simulink model "hcci_eng_with_delay"  (R2018a)
settings: Solver=VariableStepAuto  StartTime=0.0  StopTime=t_end  RelTol=1e-3
values from neighbouring files (symbols this model uses):
  A01 = f(90)    [load_param.m]
  A20 = f(70)    [load_param.m]
  A21 = f(50)    [load_param.m]
  AFR_EGO_0 = AFR_s    (= 20)    [load_param.m]
  AFR_s = 20    [load_param.m]
  alpha_1 = 0.752    [load_param.m]
  alpha_2 = -0.180    (= -0.18)    [load_param.m]
  alpha_3 = 0.015    [load_param.m]
  b1_0 = 0    [load_param.m]
  b2_0 = 0    [load_param.m]
  beta_0 = 1.035    [load_param.m]
  beta_1 = 1.1568    [load_param.m]
  dT_er2 = 75    [load_param.m]
  gamma = 1.4    [load_param.m]
  kappa_0 = -2.2107    [load_param.m]
  kappa_1 = 61.5556    [load_param.m]
  kappa_2 = 4.6052    [load_param.m]
  kappa_3 = 0.964    [load_param.m]
  m1_0 = p0*V1/(R*T1)    (= 1.2204509185e-06)    [load_param.m]
  m2_0 = p0*V2/(R*T1)    (= 1.40821259827e-05)    [load_param.m]
  N = 1000    [load_param.m]
  p0 = 101    [load_param.m]
  p2_0 = p0    (= 101)    [load_param.m]
  R = 296.25    [AR_solver_tester.m]    (also in HCCI_Combustion.m; combustion_param.m; load_param.m; testor.m)
  T1 = 90 + 273.15    (= 363.15)    [load_param.m]
  tau = 120 / N    (= 0.12)    [load_param.m]
  tau_EGO = 0.08    [load_param.m]
  u_rbl = 2    [load_param.m]
  V1 = 0.0013    [load_param.m]
  V2 = 0.015    [load_param.m]
  V_ivc = V_d + V_TDC    (= 0.000592307692308)    [AR_solver_tester.m]    (also in HCCI_Combustion.m = double(subs(Vc, theta, theta_ivc)); load_eng.m = double(subs(Vc, theta, theta_ivc)); load_param.m; testor.m = double(subs(Vc, theta, theta_ivc)))
  Wf = 11.9e-3    (= 0.0119)    [load_param.m]
undefined symbols (not defined in the file or in its folder): C_d
settings Model: Creator=Lenovo  LastModifiedBy=Lenovo

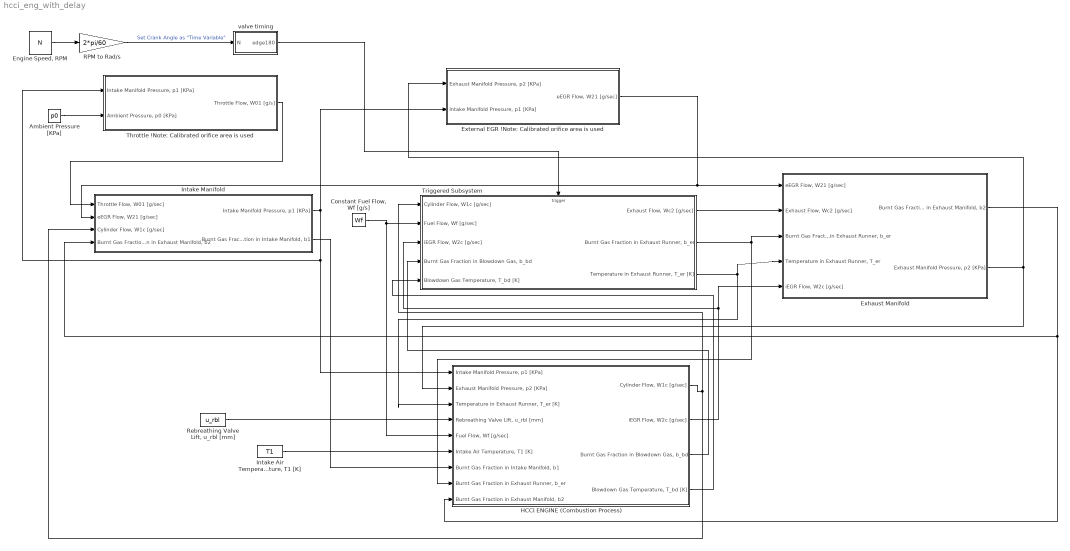
== system hcci_eng_with_delay ==
  Ambient Pressure [KPa] : Constant  Value=p0
  "Constant Fuel Flow, Wf [g/s] " : Constant  Value=Wf
  "Engine Speed, RPM" : Constant  Value=N
  Exhaust Manifold : Subsystem
  "External EGR !Note: Calibrated orifice area is used " : Subsystem
  HCCI ENGINE (Combustion Process) : Subsystem
  "Intake Air Temperature, T1 [K]" : Constant  Value=T1
  Intake Manifold : Subsystem
  RPM to Rad/s : Gain  Gain=2*pi/60
  "Rebreathing Valve Lift, u_rbl [mm]" : Constant  Value=u_rbl
  Throttle !Note: Calibrated orifice area is used : Subsystem
  Triggered Subsystem : Subsystem  TreatAsAtomicUnit=on
  valve timing : Subsystem
  wires:
  "Engine Speed, RPM"/1 -> RPM to Rad/s/1
  Ambient Pressure [KPa]/1 -> Throttle !Note: Calibrated orifice area is used/2("Ambient Pressure, p0 [KPa]")
  Throttle !Note: Calibrated orifice area is used/1("Throttle Flow, W01 [g/s]") -> Intake Manifold/1("Throttle Flow, W01 [g/sec]")
  Intake Manifold/1("Intake Manifold Pressure, p1 [KPa]") -> "External EGR !Note: Calibrated orifice area is used "/2("Intake Manifold Pressure, p1 [KPa]"), HCCI ENGINE (Combustion Process)/1("Intake Manifold Pressure, p1 [KPa]"), Throttle !Note: Calibrated orifice area is used/1("Intake Manifold Pressure, p1 [KPa]")
  "External EGR !Note: Calibrated orifice area is used "/1("eEGR Flow, W21 [g/sec]") -> Exhaust Manifold/1("eEGR Flow, W21 [g/sec]"), Intake Manifold/2("eEGR Flow, W21 [g/sec]")
  Exhaust Manifold/1("Burnt Gas Fraction in Exhaust Manifold, b2") -> HCCI ENGINE (Combustion Process)/9("Burnt Gas Fraction in Exhaust Manifold, b2"), Intake Manifold/4("Burnt Gas Fraction in Exhaust Manifold, b2")
  HCCI ENGINE (Combustion Process)/1("Cylinder Flow, W1c [g/sec]") -> Triggered Subsystem/1("Cylinder Flow, W1c [g/sec]"), Intake Manifold/3("Cylinder Flow, W1c [g/sec]")
  HCCI ENGINE (Combustion Process)/2("iEGR Flow, W2c [g/sec]") -> Exhaust Manifold/5("iEGR Flow, W2c [g/sec]"), Triggered Subsystem/3("iEGR Flow, W2c [g/sec]")
  Triggered Subsystem/1("Exhaust Flow, Wc2 [g/sec]") -> Exhaust Manifold/2("Exhaust Flow, Wc2 [g/sec]")
  Triggered Subsystem/3("Temperature in Exhaust Runner, T_er [K]") -> Exhaust Manifold/4("Temperature in Exhaust Runner, T_er"), HCCI ENGINE (Combustion Process)/3("Temperature in Exhaust Runner, T_er [K]")
  Exhaust Manifold/2("Exhaust Manifold Pressure, p2 [KPa]") -> HCCI ENGINE (Combustion Process)/2("Exhaust Manifold Pressure, p2 [KPa]"), "External EGR !Note: Calibrated orifice area is used "/1("Exhaust Manifold Pressure, p2 [KPa]")
  "Constant Fuel Flow, Wf [g/s] "/1 -> Triggered Subsystem/2("Fuel Flow, Wf [g/sec]"), HCCI ENGINE (Combustion Process)/5("Fuel Flow, Wf [g/sec] ")
  "Rebreathing Valve Lift, u_rbl [mm]"/1 -> HCCI ENGINE (Combustion Process)/4("Rebreathing Valve Lift, u_rbl [mm]")
  "Intake Air Temperature, T1 [K]"/1 -> HCCI ENGINE (Combustion Process)/6("Intake Air Temperature, T1 [K]")
  Intake Manifold/2("Burnt Gas Fraction in Intake Manifold, b1") -> HCCI ENGINE (Combustion Process)/7("Burnt Gas Fraction in Intake Manifold, b1")
  Triggered Subsystem/2("Burnt Gas Fraction in Exhaust Runner, b_er") -> Exhaust Manifold/3("Burnt Gas Fraction in Exhaust Runner, b_er"), HCCI ENGINE (Combustion Process)/8("Burnt Gas Fraction in Exhaust Runner, b_er")
  HCCI ENGINE (Combustion Process)/3("Burnt Gas Fraction in Blowdown Gas, b_bd ") -> Triggered Subsystem/4("Burnt Gas Fraction in Blowdown Gas, b_bd ")
  HCCI ENGINE (Combustion Process)/4("Blowdown Gas Temperature, T_bd [K]") -> Triggered Subsystem/5("Blowdown Gas Temperature, T_bd [K]")
  RPM to Rad/s/1 -> valve timing/1(N)  "Set Crank Angle as \"Time Variable\""
  valve timing/1(edge180) -> Triggered Subsystem/Trigger

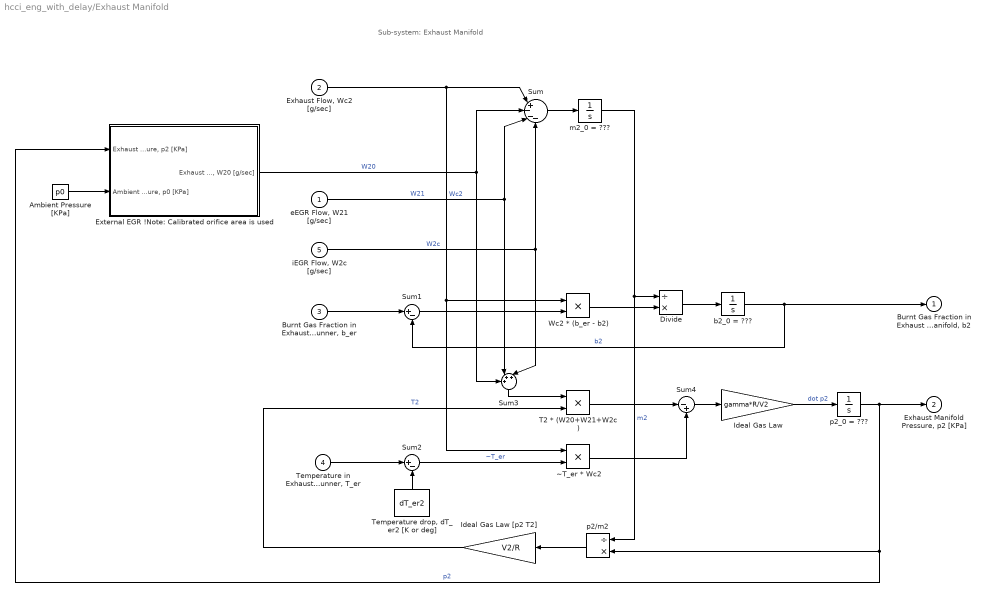
== system hcci_eng_with_delay/Exhaust Manifold ==
  note: Sub-system: Exhaust Manifold
  "eEGR Flow, W21 [g/sec]" : Inport
  "Exhaust Flow, Wc2 [g/sec]" : Inport  Port=2
  "Burnt Gas Fraction in Exhaust Runner, b_er" : Inport  Port=3
  "Temperature in Exhaust Runner, T_er" : Inport  Port=4
  "iEGR Flow, W2c [g/sec]" : Inport  Port=5
  Ambient Pressure [KPa] : Constant  Value=p0
  Divide : Product  Inputs=/*
  "External EGR !Note: Calibrated orifice area is used " : Subsystem
  Ideal Gas Law : Gain  Gain=gamma*R/V2
  Ideal Gas Law [p2 T2] : Gain  Gain=V2/R
  Sum : Sum  Inputs=|+---
  Sum1 : Sum  Inputs=|+-
  Sum2 : Sum  Inputs=|+-
  Sum3 : Sum  Inputs=+++|
  Sum4 : Sum  Inputs=|-+
  T2 * (W20+W21+W2c) : Product
  "Temperature drop, dT_er2 [K or deg] " : Constant  Value=dT_er2
  Wc2 * (b_er - b2) : Product
  b2_0 = ??? : Integrator  InitialCondition=b2_0
  m2_0 = ??? : Integrator  InitialCondition=m2_0
  p2/m2 : Product  Inputs=/*
  p2_0 = ??? : Integrator  InitialCondition=p2_0
  ~T_er * Wc2 : Product
  "Burnt Gas Fraction in Exhaust Manifold, b2" : Outport
  "Exhaust Manifold Pressure, p2 [KPa]" : Outport  Port=2
  wires:
  "Exhaust Flow, Wc2 [g/sec]"/1 -> Sum/1, Wc2 * (b_er - b2)/1, ~T_er * Wc2/1  "Wc2"
  "External EGR !Note: Calibrated orifice area is used "/1("Exhaust Flow, W20 [g/sec]") -> Sum/2, Sum3/1  "W20"
  "eEGR Flow, W21 [g/sec]"/1 -> Sum3/2, Sum/3  "W21"
  "iEGR Flow, W2c [g/sec]"/1 -> Sum3/3, Sum/4  "W2c"
  Sum/1 -> m2_0 = ???/1
  m2_0 = ???/1 -> p2/m2/1, Divide/1  "m2"
  Divide/1 -> b2_0 = ???/1
  Wc2 * (b_er - b2)/1 -> Divide/2
  b2_0 = ???/1 -> "Burnt Gas Fraction in Exhaust Manifold, b2"/1, Sum1/2  "b2"
  "Burnt Gas Fraction in Exhaust Runner, b_er"/1 -> Sum1/1
  Sum1/1 -> Wc2 * (b_er - b2)/2
  "Temperature in Exhaust Runner, T_er"/1 -> Sum2/1
  "Temperature drop, dT_er2 [K or deg] "/1 -> Sum2/2
  Sum2/1 -> ~T_er * Wc2/2  "~T_er"
  Sum3/1 -> T2 * (W20+W21+W2c)/1
  Ideal Gas Law [p2 T2]/1 -> T2 * (W20+W21+W2c)/2  "T2"
  T2 * (W20+W21+W2c)/1 -> Sum4/1
  ~T_er * Wc2/1 -> Sum4/2
  Sum4/1 -> Ideal Gas Law/1
  Ideal Gas Law/1 -> p2_0 = ???/1  "dot p2"
  p2_0 = ???/1 -> "Exhaust Manifold Pressure, p2 [KPa]"/1, "External EGR !Note: Calibrated orifice area is used "/1("Exhaust Manifold Pressure, p2 [KPa]"), p2/m2/2  "p2"
  p2/m2/1 -> Ideal Gas Law [p2 T2]/1
  Ambient Pressure [KPa]/1 -> "External EGR !Note: Calibrated orifice area is used "/2("Ambient Pressure, p0 [KPa]")

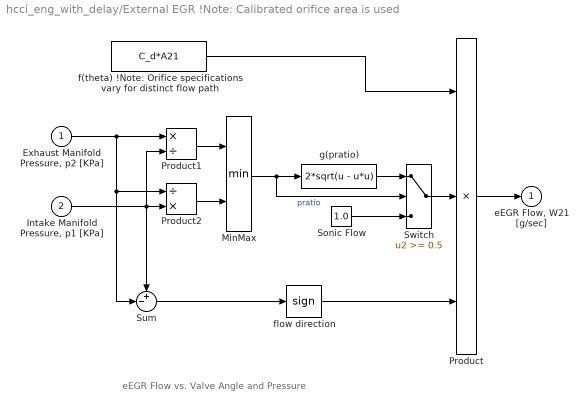
== system hcci_eng_with_delay/External EGR !Note: Calibrated orifice area is used  ==
  note: eEGR Flow vs. Valve Angle and Pressure
  "Exhaust Manifold Pressure, p2 [KPa]" : Inport
  "Intake Manifold Pressure, p1 [KPa]" : Inport  Port=2
  MinMax : MinMax  Inputs=2  SaturateOnIntegerOverflow=on  InputSameDT=on
  Product : Product  Inputs=3  SaturateOnIntegerOverflow=on  RndMeth=Zero  InputSameDT=on  OutDataTypeStr=Inherit: Same as first input
  Product1 : Product  Inputs=*/  SaturateOnIntegerOverflow=on  RndMeth=Zero  InputSameDT=on  OutDataTypeStr=Inherit: Same as first input
  Product2 : Product  Inputs=/*  SaturateOnIntegerOverflow=on  RndMeth=Zero  InputSameDT=on  OutDataTypeStr=Inherit: Same as first input
  "Sonic Flow " : Constant  Value=1.0
  Sum : Sum  Inputs=+-|  SaturateOnIntegerOverflow=on  InputSameDT=on  OutDataTypeStr=Inherit: Same as first input
  Switch : Switch  Threshold=0.5  SaturateOnIntegerOverflow=on  InputSameDT=on
  "f(theta) !Note: Orifice specifications vary for distinct flow path " : Constant  Value=C_d*A21
  flow direction : Signum
  g(pratio) : Fcn  Expr=2*sqrt(u - u*u)
  "eEGR Flow, W21 [g/sec]" : Outport  InitialOutput=0
  wires:
  "Exhaust Manifold Pressure, p2 [KPa]"/1 -> Sum/2, Product2/1, Product1/1
  Product2/1 -> MinMax/2
  Product1/1 -> MinMax/1
  "Intake Manifold Pressure, p1 [KPa]"/1 -> Sum/1, Product2/2, Product1/2
  g(pratio)/1 -> Switch/1
  "Sonic Flow "/1 -> Switch/3
  Switch/1 -> Product/2
  flow direction/1 -> Product/3
  Sum/1 -> flow direction/1
  MinMax/1 -> Switch/2, g(pratio)/1  "pratio"
  Product/1 -> "eEGR Flow, W21 [g/sec]"/1
  "f(theta) !Note: Orifice specifications vary for distinct flow path "/1 -> Product/1

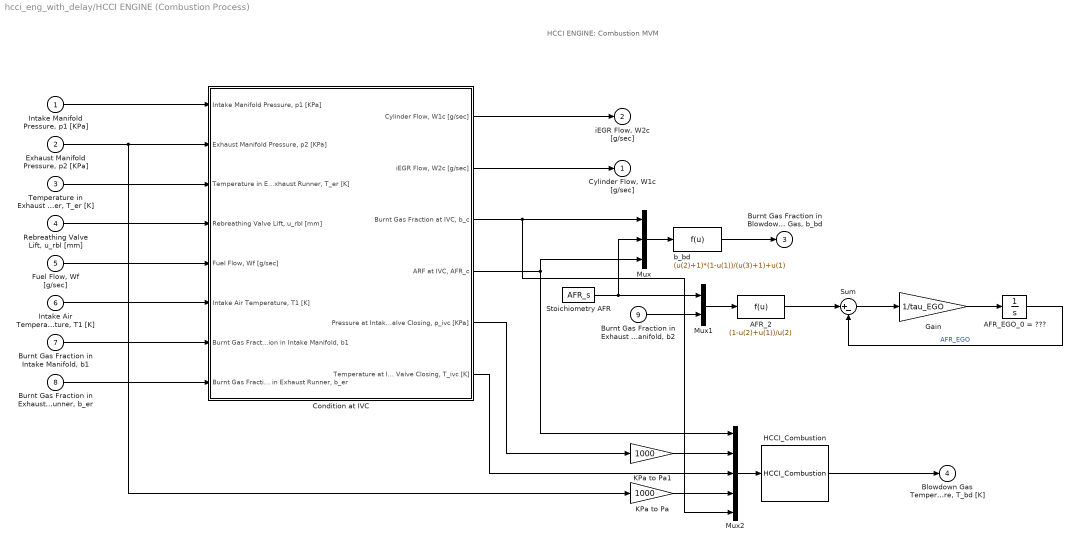
== system hcci_eng_with_delay/HCCI ENGINE (Combustion Process) ==
  note: HCCI ENGINE: Combustion MVM
  "Intake Manifold Pressure, p1 [KPa]" : Inport
  "Exhaust Manifold Pressure, p2 [KPa]" : Inport  Port=2
  "Temperature in Exhaust Runner, T_er [K]" : Inport  Port=3
  "Rebreathing Valve Lift, u_rbl [mm]" : Inport  Port=4
  "Fuel Flow, Wf [g/sec] " : Inport  Port=5
  "Intake Air Temperature, T1 [K]" : Inport  Port=6
  "Burnt Gas Fraction in Intake Manifold, b1" : Inport  Port=7
  "Burnt Gas Fraction in Exhaust Runner, b_er" : Inport  Port=8
  "Burnt Gas Fraction in Exhaust Manifold, b2" : Inport  Port=9
  AFR_2 : Fcn  Expr=(1-u(2)+u(1))/u(2)
  AFR_EGO_0 = ??? : Integrator  InitialCondition=AFR_EGO_0
  Condition at IVC : Subsystem
  Gain : Gain  Gain=1/tau_EGO
  HCCI_Combustion : MATLABFcn  MATLABFcn=HCCI_Combustion
  KPa to Pa : Gain  Gain=1000
  KPa to Pa1 : Gain  Gain=1000
  Mux : Mux  Inputs=3
  Mux1 : Mux  Inputs=2
  Mux2 : Mux  Inputs=5
  Stoichiometry AFR : Constant  Value=AFR_s
  Sum : Sum  Inputs=|+-
  b_bd : Fcn  Expr=(u(2)+1)*(1-u(1))/(u(3)+1)+u(1)
  "Cylinder Flow, W1c [g/sec]" : Outport
  "iEGR Flow, W2c [g/sec]" : Outport  Port=2
  "Burnt Gas Fraction in Blowdown Gas, b_bd " : Outport  Port=3
  "Blowdown Gas Temperature, T_bd [K]" : Outport  Port=4
  wires:
  "Intake Manifold Pressure, p1 [KPa]"/1 -> Condition at IVC/1("Intake Manifold Pressure, p1 [KPa]")
  "Exhaust Manifold Pressure, p2 [KPa]"/1 -> KPa to Pa/1, Condition at IVC/2("Exhaust Manifold Pressure, p2 [KPa]")
  "Temperature in Exhaust Runner, T_er [K]"/1 -> Condition at IVC/3("Temperature in Exhaust Runner, T_er [K]")
  "Rebreathing Valve Lift, u_rbl [mm]"/1 -> Condition at IVC/4("Rebreathing Valve Lift, u_rbl [mm]")
  "Fuel Flow, Wf [g/sec] "/1 -> Condition at IVC/5("Fuel Flow, Wf [g/sec] ")
  "Intake Air Temperature, T1 [K]"/1 -> Condition at IVC/6("Intake Air Temperature, T1 [K]")
  Condition at IVC/1("Cylinder Flow, W1c [g/sec]") -> "iEGR Flow, W2c [g/sec]"/1
  Condition at IVC/2("iEGR Flow, W2c [g/sec]") -> "Cylinder Flow, W1c [g/sec]"/1
  "Burnt Gas Fraction in Intake Manifold, b1"/1 -> Condition at IVC/7("Burnt Gas Fraction in Intake Manifold, b1")
  "Burnt Gas Fraction in Exhaust Runner, b_er"/1 -> Condition at IVC/8("Burnt Gas Fraction in Exhaust Runner, b_er")
  Stoichiometry AFR/1 -> Mux1/1, Mux/2
  Condition at IVC/3("Burnt Gas Fraction at IVC, b_c") -> Mux2/5, Mux/1
  Condition at IVC/4("ARF at IVC, AFR_c") -> Mux2/1, Mux/3
  Mux/1 -> b_bd/1
  b_bd/1 -> "Burnt Gas Fraction in Blowdown Gas, b_bd "/1
  "Burnt Gas Fraction in Exhaust Manifold, b2"/1 -> Mux1/2
  Mux1/1 -> AFR_2/1
  AFR_2/1 -> Sum/1
  Sum/1 -> Gain/1
  Gain/1 -> AFR_EGO_0 = ???/1
  AFR_EGO_0 = ???/1 -> Sum/2  "AFR_EGO"
  HCCI_Combustion/1 -> "Blowdown Gas Temperature, T_bd [K]"/1
  Condition at IVC/5("Pressure at Intake Valve Closing, p_ivc [KPa]") -> KPa to Pa1/1
  Condition at IVC/6("Temperature at Intake Valve Closing, T_ivc [K]") -> Mux2/3
  KPa to Pa1/1 -> Mux2/2
  KPa to Pa/1 -> Mux2/4
  Mux2/1 -> HCCI_Combustion/1

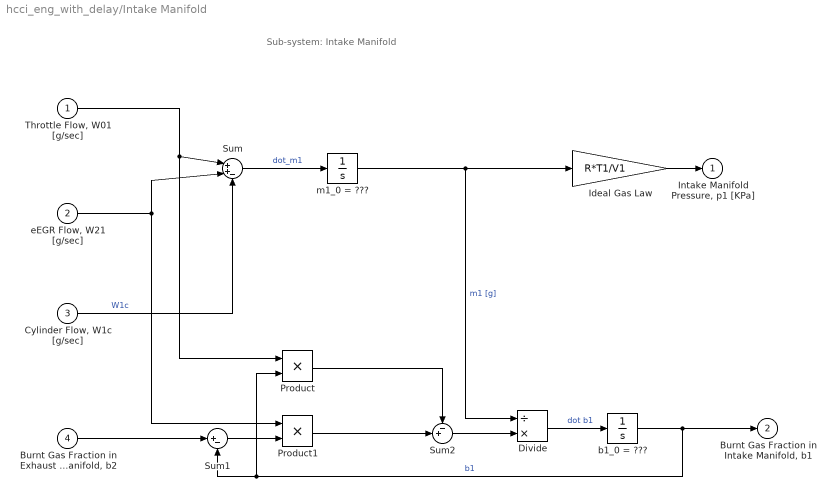
== system hcci_eng_with_delay/Intake Manifold ==
  note: Sub-system: Intake Manifold
  "Throttle Flow, W01 [g/sec]" : Inport
  "eEGR Flow, W21 [g/sec]" : Inport  Port=2
  "Cylinder Flow, W1c [g/sec]" : Inport  Port=3
  "Burnt Gas Fraction in Exhaust Manifold, b2" : Inport  Port=4
  Divide : Product  Inputs=/*
  Ideal Gas Law : Gain  Gain=R*T1/V1
  Product : Product
  Product1 : Product
  Sum : Sum  Inputs=|++-
  Sum1 : Sum  Inputs=|+-
  Sum2 : Sum  Inputs=-+|
  b1_0 = ??? : Integrator  InitialCondition=b1_0
  m1_0 = ??? : Integrator  InitialCondition=m1_0
  "Intake Manifold Pressure, p1 [KPa]" : Outport
  "Burnt Gas Fraction in Intake Manifold, b1" : Outport  Port=2
  wires:
  "Cylinder Flow, W1c [g/sec]"/1 -> Sum/3  "W1c"
  "Throttle Flow, W01 [g/sec]"/1 -> Product/1, Sum/1
  "eEGR Flow, W21 [g/sec]"/1 -> Product1/1, Sum/2
  Sum/1 -> m1_0 = ???/1  "dot_m1"
  m1_0 = ???/1 -> Ideal Gas Law/1, Divide/1  "m1 [g]"
  "Burnt Gas Fraction in Exhaust Manifold, b2"/1 -> Sum1/1
  Sum1/1 -> Product1/2
  Product1/1 -> Sum2/2
  Product/1 -> Sum2/1
  Sum2/1 -> Divide/2
  Divide/1 -> b1_0 = ???/1  "dot b1"
  b1_0 = ???/1 -> Product/2, Sum1/2, "Burnt Gas Fraction in Intake Manifold, b1"/1  "b1"
  Ideal Gas Law/1 -> "Intake Manifold Pressure, p1 [KPa]"/1

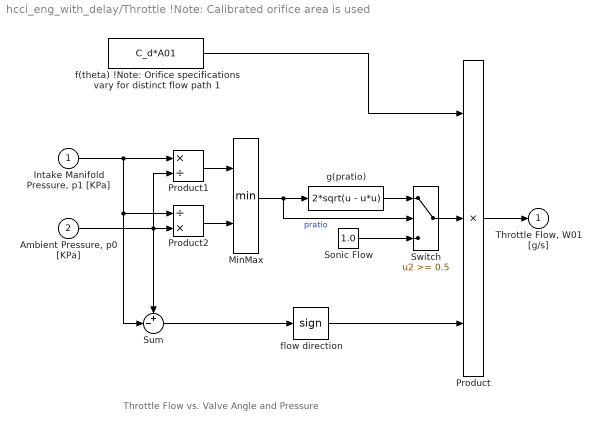
== system hcci_eng_with_delay/Throttle !Note: Calibrated orifice area is used ==
  note: Throttle Flow vs. Valve Angle and Pressure
  "Intake Manifold Pressure, p1 [KPa]" : Inport
  "Ambient Pressure, p0 [KPa]" : Inport  Port=2
  MinMax : MinMax  Inputs=2  SaturateOnIntegerOverflow=on  InputSameDT=on
  Product : Product  Inputs=3  SaturateOnIntegerOverflow=on  RndMeth=Zero  InputSameDT=on  OutDataTypeStr=Inherit: Same as first input
  Product1 : Product  Inputs=*/  SaturateOnIntegerOverflow=on  RndMeth=Zero  InputSameDT=on  OutDataTypeStr=Inherit: Same as first input
  Product2 : Product  Inputs=/*  SaturateOnIntegerOverflow=on  RndMeth=Zero  InputSameDT=on  OutDataTypeStr=Inherit: Same as first input
  "Sonic Flow " : Constant  Value=1.0
  Sum : Sum  Inputs=+-|  SaturateOnIntegerOverflow=on  InputSameDT=on  OutDataTypeStr=Inherit: Same as first input
  Switch : Switch  Threshold=0.5  SaturateOnIntegerOverflow=on  InputSameDT=on
  f(theta) !Note: Orifice specifications vary for distinct flow path 1 : Constant  Value=C_d*A01
  flow direction : Signum
  g(pratio) : Fcn  Expr=2*sqrt(u - u*u)
  "Throttle Flow, W01 [g/s]" : Outport  InitialOutput=0
  wires:
  "Intake Manifold Pressure, p1 [KPa]"/1 -> Sum/2, Product2/1, Product1/1
  Product2/1 -> MinMax/2
  Product1/1 -> MinMax/1
  "Ambient Pressure, p0 [KPa]"/1 -> Sum/1, Product2/2, Product1/2
  g(pratio)/1 -> Switch/1
  "Sonic Flow "/1 -> Switch/3
  Switch/1 -> Product/2
  flow direction/1 -> Product/3
  Sum/1 -> flow direction/1
  MinMax/1 -> Switch/2, g(pratio)/1  "pratio"
  Product/1 -> "Throttle Flow, W01 [g/s]"/1
  f(theta) !Note: Orifice specifications vary for distinct flow path 1/1 -> Product/1

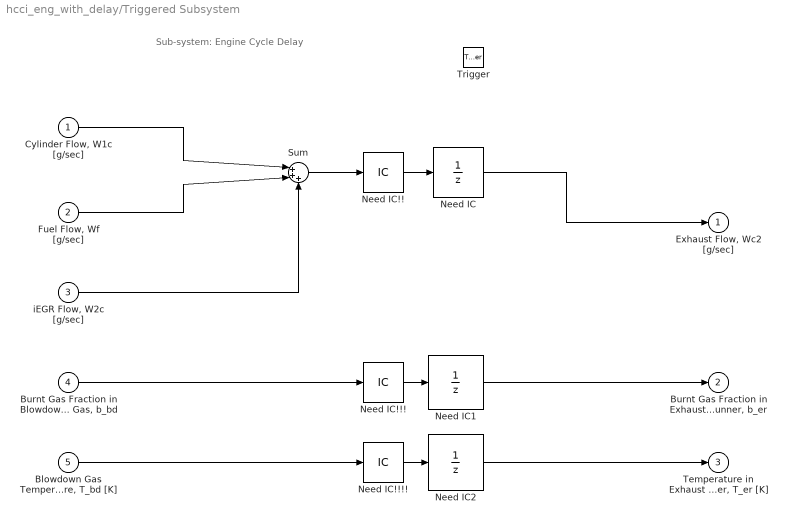
== system hcci_eng_with_delay/Triggered Subsystem ==
  note: Sub-system: Engine Cycle Delay
  "Cylinder Flow, W1c [g/sec]" : Inport
  "Fuel Flow, Wf [g/sec]" : Inport  Port=2
  "iEGR Flow, W2c [g/sec]" : Inport  Port=3
  "Burnt Gas Fraction in Blowdown Gas, b_bd " : Inport  Port=4
  "Blowdown Gas Temperature, T_bd [K]" : Inport  Port=5
  Trigger : TriggerPort  VariantControl=Variant
  Need IC : UnitDelay  SampleTime=-1
  Need IC!! : InitialCondition  Value=0.156
  Need IC!!! : InitialCondition  Value=0.156
  Need IC!!!! : InitialCondition  Value=0.156
  Need IC1 : UnitDelay  SampleTime=-1
  Need IC2 : UnitDelay  SampleTime=-1
  Sum : Sum  Inputs=|+++
  "Exhaust Flow, Wc2 [g/sec]" : Outport
  "Burnt Gas Fraction in Exhaust Runner, b_er" : Outport  Port=2
  "Temperature in Exhaust Runner, T_er [K]" : Outport  Port=3
  wires:
  Need IC2/1 -> "Temperature in Exhaust Runner, T_er [K]"/1
  "Burnt Gas Fraction in Blowdown Gas, b_bd "/1 -> Need IC!!!/1
  "Blowdown Gas Temperature, T_bd [K]"/1 -> Need IC!!!!/1
  "iEGR Flow, W2c [g/sec]"/1 -> Sum/3
  "Fuel Flow, Wf [g/sec]"/1 -> Sum/2
  Need IC/1 -> "Exhaust Flow, Wc2 [g/sec]"/1
  Need IC1/1 -> "Burnt Gas Fraction in Exhaust Runner, b_er"/1
  "Cylinder Flow, W1c [g/sec]"/1 -> Sum/1
  Sum/1 -> Need IC!!/1
  Need IC!!/1 -> Need IC/1
  Need IC!!!/1 -> Need IC1/1
  Need IC!!!!/1 -> Need IC2/1

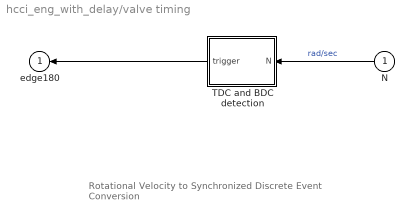
== system hcci_eng_with_delay/valve timing ==
  note: Rotational Velocity to Synchronized
      | Discrete Event Conversion
  N : Inport
  TDC and BDC detection : Subsystem
  edge180 : Outport  InitialOutput=-1
  wires:
  N/1 -> TDC and BDC detection/1(N)  "rad/sec"
  TDC and BDC detection/1(trigger) -> edge180/1

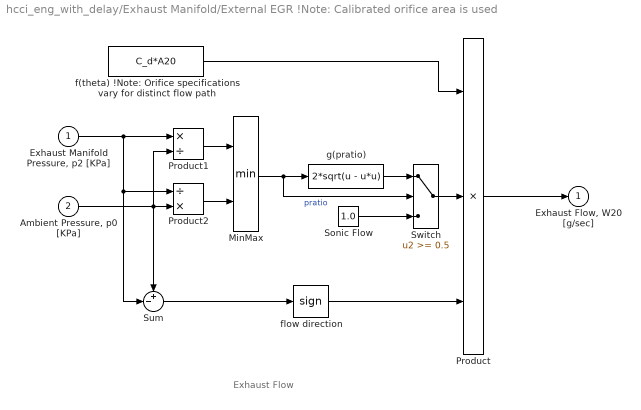
== system hcci_eng_with_delay/Exhaust Manifold/External EGR !Note: Calibrated orifice area is used  ==
  note: Exhaust Flow
  "Exhaust Manifold Pressure, p2 [KPa]" : Inport
  "Ambient Pressure, p0 [KPa]" : Inport  Port=2
  MinMax : MinMax  Inputs=2  SaturateOnIntegerOverflow=on  InputSameDT=on
  Product : Product  Inputs=3  SaturateOnIntegerOverflow=on  RndMeth=Zero  InputSameDT=on  OutDataTypeStr=Inherit: Same as first input
  Product1 : Product  Inputs=*/  SaturateOnIntegerOverflow=on  RndMeth=Zero  InputSameDT=on  OutDataTypeStr=Inherit: Same as first input
  Product2 : Product  Inputs=/*  SaturateOnIntegerOverflow=on  RndMeth=Zero  InputSameDT=on  OutDataTypeStr=Inherit: Same as first input
  "Sonic Flow " : Constant  Value=1.0
  Sum : Sum  Inputs=+-|  SaturateOnIntegerOverflow=on  InputSameDT=on  OutDataTypeStr=Inherit: Same as first input
  Switch : Switch  Threshold=0.5  SaturateOnIntegerOverflow=on  InputSameDT=on
  "f(theta) !Note: Orifice specifications vary for distinct flow path " : Constant  Value=C_d*A20
  flow direction : Signum
  g(pratio) : Fcn  Expr=2*sqrt(u - u*u)
  "Exhaust Flow, W20 [g/sec]" : Outport  InitialOutput=0
  wires:
  "Exhaust Manifold Pressure, p2 [KPa]"/1 -> Sum/2, Product2/1, Product1/1
  Product2/1 -> MinMax/2
  Product1/1 -> MinMax/1
  "Ambient Pressure, p0 [KPa]"/1 -> Sum/1, Product2/2, Product1/2
  g(pratio)/1 -> Switch/1
  "Sonic Flow "/1 -> Switch/3
  Switch/1 -> Product/2
  flow direction/1 -> Product/3
  Sum/1 -> flow direction/1
  MinMax/1 -> Switch/2, g(pratio)/1  "pratio"
  Product/1 -> "Exhaust Flow, W20 [g/sec]"/1
  "f(theta) !Note: Orifice specifications vary for distinct flow path "/1 -> Product/1

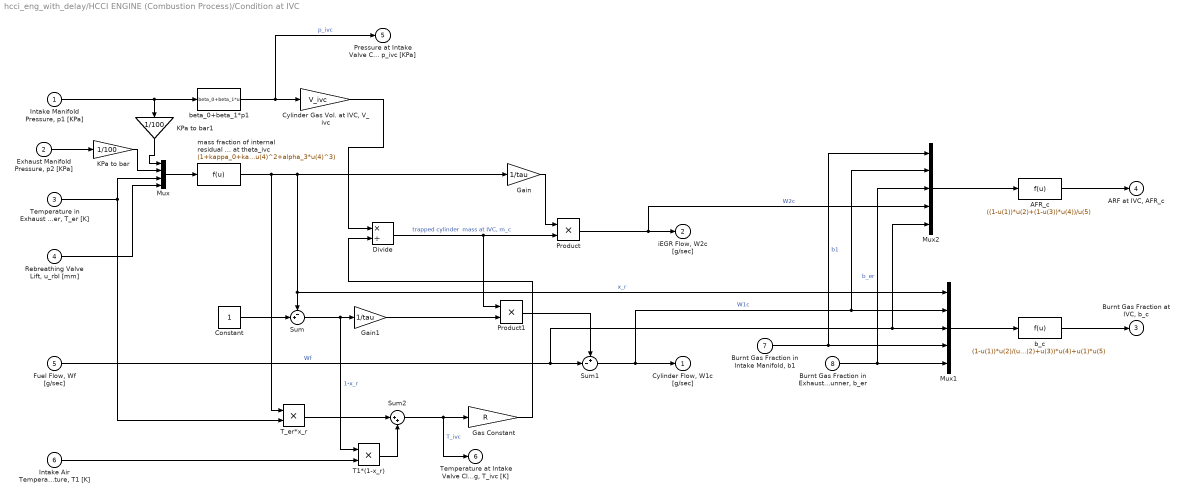
== system hcci_eng_with_delay/HCCI ENGINE (Combustion Process)/Condition at IVC ==
  "Intake Manifold Pressure, p1 [KPa]" : Inport
  "Exhaust Manifold Pressure, p2 [KPa]" : Inport  Port=2
  "Temperature in Exhaust Runner, T_er [K]" : Inport  Port=3
  "Rebreathing Valve Lift, u_rbl [mm]" : Inport  Port=4
  "Fuel Flow, Wf [g/sec] " : Inport  Port=5
  "Intake Air Temperature, T1 [K]" : Inport  Port=6
  "Burnt Gas Fraction in Intake Manifold, b1" : Inport  Port=7
  "Burnt Gas Fraction in Exhaust Runner, b_er" : Inport  Port=8
  AFR_c : Fcn  Expr=((1-u(1))*u(2)+(1-u(3))*u(4))/u(5)
  Constant : Constant
  "Cylinder Gas Vol. at IVC, V_ivc" : Gain  Gain=V_ivc
  Divide : Product  Inputs=*/
  Gain : Gain  Gain=1/tau
  Gain1 : Gain  Gain=1/tau
  Gas Constant : Gain  Gain=R
  KPa to bar : Gain  Gain=1/100
  KPa to bar1 : Gain  Gain=1/100
  Mux : Mux
  Mux1 : Mux  Inputs=5
  Mux2 : Mux  Inputs=5
  Product : Product
  Product1 : Product
  Sum : Sum  Inputs=-+|
  Sum1 : Sum  Inputs=+-|
  Sum2 : Sum  Inputs=|++
  T1*(1-x_r) : Product
  "T_er*x_r " : Product
  b_c : Fcn  Expr=(1-u(1))*u(2)/(u(2)+u(3))*u(4)+u(1)*u(5)
  beta_0+beta_1*p1 : Fcn  Expr=beta_0+beta_1*u
  mass fraction of internal residual gases at theta_ivc : Fcn  Expr=(1+kappa_0+kappa_1*u(1)^kappa_3/(u(2)^kappa_2*sqrt(u(3))))*(alpha_1*u(4)+alpha_2*u(4)^2+alpha_3*u(4)^3)
  "Cylinder Flow, W1c [g/sec]" : Outport
  "iEGR Flow, W2c [g/sec]" : Outport  Port=2
  "Burnt Gas Fraction at IVC, b_c" : Outport  Port=3
  "ARF at IVC, AFR_c" : Outport  Port=4
  "Pressure at Intake Valve Closing, p_ivc [KPa]" : Outport  Port=5
  "Temperature at Intake Valve Closing, T_ivc [K]" : Outport  Port=6
  wires:
  "T_er*x_r "/1 -> Sum2/1
  beta_0+beta_1*p1/1 -> "Pressure at Intake Valve Closing, p_ivc [KPa]"/1, "Cylinder Gas Vol. at IVC, V_ivc"/1  "p_ivc"
  Gas Constant/1 -> Divide/2
  Sum2/1 -> "Temperature at Intake Valve Closing, T_ivc [K]"/1, Gas Constant/1  "T_ivc"
  T1*(1-x_r)/1 -> Sum2/2
  Mux/1 -> mass fraction of internal residual gases at theta_ivc/1
  Product1/1 -> Sum1/1
  Product/1 -> Mux2/4, "iEGR Flow, W2c [g/sec]"/1  "W2c"
  "Temperature in Exhaust Runner, T_er [K]"/1 -> "T_er*x_r "/2, Mux/3
  "Intake Manifold Pressure, p1 [KPa]"/1 -> beta_0+beta_1*p1/1, KPa to bar1/1
  Sum/1 -> Gain1/1, T1*(1-x_r)/1  "1-x_r"
  "Cylinder Gas Vol. at IVC, V_ivc"/1 -> Divide/1
  Divide/1 -> Product/2, Product1/1  "trapped cylinder  mass at IVC, m_c"
  "Exhaust Manifold Pressure, p2 [KPa]"/1 -> KPa to bar/1
  Constant/1 -> Sum/2
  Gain1/1 -> Product1/2
  "Intake Air Temperature, T1 [K]"/1 -> T1*(1-x_r)/2
  "Rebreathing Valve Lift, u_rbl [mm]"/1 -> Mux/4
  "Fuel Flow, Wf [g/sec] "/1 -> Mux2/5, Mux1/3, Sum1/2  "Wf"
  Gain/1 -> Product/1
  Sum1/1 -> Mux1/2, Mux2/2, "Cylinder Flow, W1c [g/sec]"/1  "W1c"
  mass fraction of internal residual gases at theta_ivc/1 -> Gain/1, Mux1/1, Sum/1, "T_er*x_r "/1  "x_r"
  "Burnt Gas Fraction in Intake Manifold, b1"/1 -> Mux1/4, Mux2/1  "b1"
  Mux1/1 -> b_c/1
  b_c/1 -> "Burnt Gas Fraction at IVC, b_c"/1
  AFR_c/1 -> "ARF at IVC, AFR_c"/1
  Mux2/1 -> AFR_c/1
  "Burnt Gas Fraction in Exhaust Runner, b_er"/1 -> Mux2/3, Mux1/5  "b_er"
  KPa to bar1/1 -> Mux/1
  KPa to bar/1 -> Mux/2

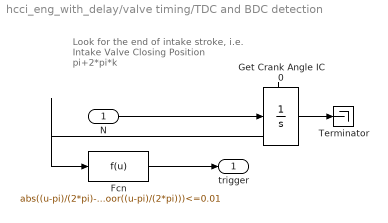
== system hcci_eng_with_delay/valve timing/TDC and BDC detection ==
  note: Look for the end of intake stroke, i.e. Intake Valve Closing Position pi+2*pi*k
  N : Inport
  Fcn : Fcn  Expr=abs((u-pi)/(2*pi)-floor((u-pi)/(2*pi)))<=0.01
  Get Crank Angle IC 0 : Integrator  ShowStatePort=on
  Terminator : Terminator
  trigger : Outport  InitialOutput=0
  wires:
  N/1 -> Get Crank Angle IC 0/1
  Fcn/1 -> trigger/1
  Get Crank Angle IC 0/State -> Fcn/1
  Get Crank Angle IC 0/1 -> Terminator/1
